simulink model "teleoperationTwoArm"  (R2012b)
settings: Solver=ode45  StartTime=0.0  StopTime=10  RelTol=1e-3
settings Model: Creator=aruszkowski  LastModifiedBy=davinci
settings DataIOCC: SignalLoggingSaveFormat=ModelDataLogs  SaveOutput=off  SaveTime=off
settings OptimizationCC: ExpressionDepthLimit=128
settings DebuggingCC: ReadBeforeWriteMsg=DisableAll  WriteAfterWriteMsg=DisableAll  WriteAfterReadMsg=DisableAll  MultiTaskDSMMsg=warning  MultiTaskCondExecSysMsg=none  StateNameClashWarn=none  StrictBusMsg=None
settings ModelReferenceCC: UpdateModelReferenceTargets=IfOutOfDate
settings SFSimCC: SFSimEcho=off
settings RTWCC: IncludeERTFirstTime=on
settings CodeAppCC: CustomSymbolStrType=$N$R$M_T  InternalIdentifier=Shortened

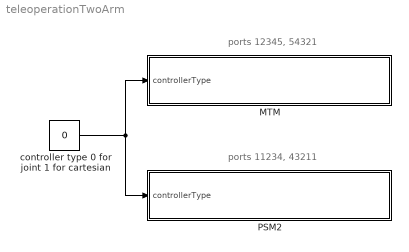
== system teleoperationTwoArm ==
  note: ports 12345, 54321
  note: ports 11234, 43211
  MTM : Subsystem
  PSM2 : Subsystem
  controller type 0 for joint 1 for cartesian : Constant  Value=0
  wires:
  controller type 0 for joint 1 for cartesian/1 -> PSM2/1(controllerType), MTM/1(controllerType)

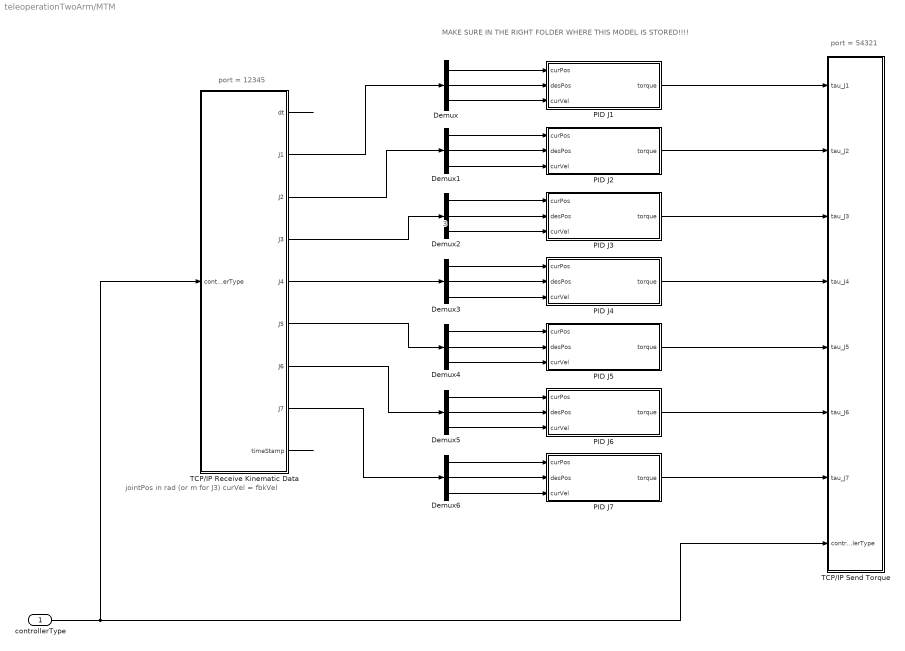
== system teleoperationTwoArm/MTM ==
  note: MAKE SURE IN THE RIGHT FOLDER WHERE THIS MODEL IS STORED!!!!
  note: port = 54321
  note: port = 12345
  note: 3
  note: jointPos in rad (or m for J3)
      | curVel = fbkVel
  controllerType : Inport
  Demux{,1..6} (7 alike) : Demux  Outputs=3
  PID J1 : Subsystem
  PID J2 : Subsystem
  PID J3 : Subsystem
  PID J4 : Subsystem
  PID J5 : Subsystem
  PID J6 : Subsystem
  PID J7 : Subsystem
  TCP/IP Receive Kinematic Data : Subsystem
  TCP/IP Send Torque : Subsystem  TreatAsAtomicUnit=on
  wires:
  TCP/IP Receive Kinematic Data/8(J7) -> Demux6/1
  Demux/1 -> PID J1/1(curPos)
  Demux/2 -> PID J1/2(desPos)
  Demux1/2 -> PID J2/2(desPos)
  Demux1/3 -> PID J2/3(curVel)
  Demux2/1 -> PID J3/1(curPos)
  PID J5/1(torque) -> TCP/IP Send Torque/5(tau_J5)
  PID J7/1(torque) -> TCP/IP Send Torque/7(tau_J7)
  controllerType/1 -> TCP/IP Receive Kinematic Data/1(controllerType), TCP/IP Send Torque/8(controllerType)
  TCP/IP Receive Kinematic Data/6(J5) -> Demux4/1
  TCP/IP Receive Kinematic Data/7(J6) -> Demux5/1
  Demux5/3 -> PID J6/3(curVel)
  Demux6/1 -> PID J7/1(curPos)
  TCP/IP Receive Kinematic Data/1(dt) -> ?
  TCP/IP Receive Kinematic Data/9(timeStamp) -> ?
  Demux6/2 -> PID J7/2(desPos)
  Demux4/3 -> PID J5/3(curVel)
  TCP/IP Receive Kinematic Data/2(J1) -> Demux/1
  Demux1/1 -> PID J2/1(curPos)
  Demux2/3 -> PID J3/3(curVel)
  Demux2/2 -> PID J3/2(desPos)
  TCP/IP Receive Kinematic Data/3(J2) -> Demux1/1
  Demux4/2 -> PID J5/2(desPos)
  Demux5/1 -> PID J6/1(curPos)
  Demux/3 -> PID J1/3(curVel)
  Demux5/2 -> PID J6/2(desPos)
  TCP/IP Receive Kinematic Data/4(J3) -> Demux2/1
  TCP/IP Receive Kinematic Data/5(J4) -> Demux3/1
  PID J2/1(torque) -> TCP/IP Send Torque/2(tau_J2)
  PID J4/1(torque) -> TCP/IP Send Torque/4(tau_J4)
  PID J3/1(torque) -> TCP/IP Send Torque/3(tau_J3)
  PID J1/1(torque) -> TCP/IP Send Torque/1(tau_J1)
  Demux6/3 -> PID J7/3(curVel)
  PID J6/1(torque) -> TCP/IP Send Torque/6(tau_J6)
  Demux3/3 -> PID J4/3(curVel)
  Demux4/1 -> PID J5/1(curPos)
  Demux3/1 -> PID J4/1(curPos)
  Demux3/2 -> PID J4/2(desPos)

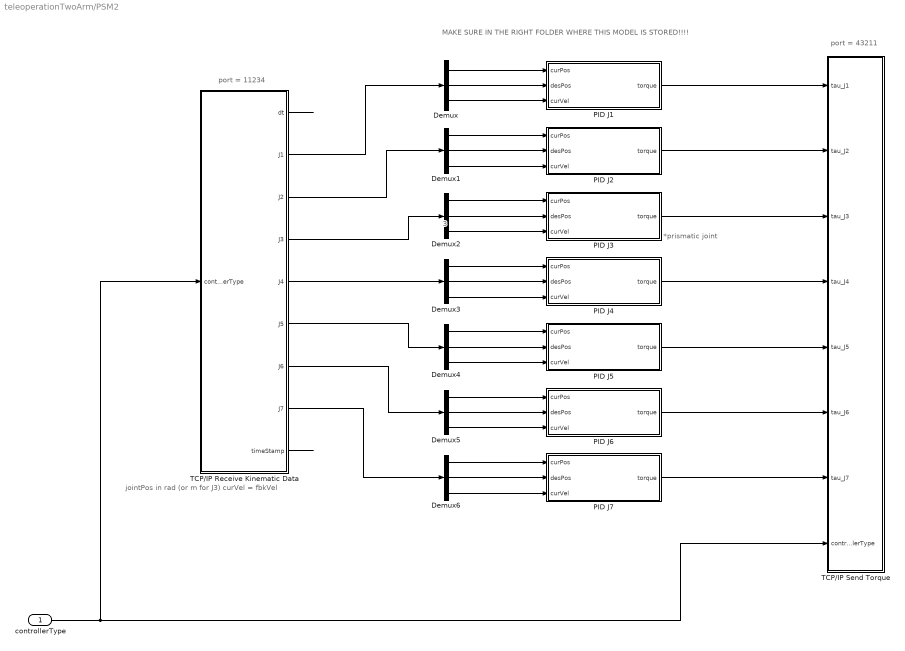
== system teleoperationTwoArm/PSM2 ==
  note: *prismatic joint
  note: jointPos in rad (or m for J3)
      | curVel = fbkVel
  note: 3
  note: port = 11234
  note: port = 43211
  note: MAKE SURE IN THE RIGHT FOLDER WHERE THIS MODEL IS STORED!!!!
  controllerType : Inport
  Demux{,1..6} (7 alike) : Demux  Outputs=3
  PID J1 : Subsystem
  PID J2 : Subsystem
  PID J3 : Subsystem
  PID J4 : Subsystem
  PID J5 : Subsystem
  PID J6 : Subsystem
  PID J7 : Subsystem
  TCP/IP Receive Kinematic Data : Subsystem
  TCP/IP Send Torque : Subsystem  TreatAsAtomicUnit=on
  wires:
  Demux3/2 -> PID J4/2(desPos)
  Demux3/1 -> PID J4/1(curPos)
  Demux4/1 -> PID J5/1(curPos)
  Demux3/3 -> PID J4/3(curVel)
  PID J6/1(torque) -> TCP/IP Send Torque/6(tau_J6)
  Demux6/3 -> PID J7/3(curVel)
  PID J1/1(torque) -> TCP/IP Send Torque/1(tau_J1)
  PID J3/1(torque) -> TCP/IP Send Torque/3(tau_J3)
  PID J4/1(torque) -> TCP/IP Send Torque/4(tau_J4)
  PID J2/1(torque) -> TCP/IP Send Torque/2(tau_J2)
  TCP/IP Receive Kinematic Data/5(J4) -> Demux3/1
  TCP/IP Receive Kinematic Data/4(J3) -> Demux2/1
  Demux5/2 -> PID J6/2(desPos)
  Demux/3 -> PID J1/3(curVel)
  Demux5/1 -> PID J6/1(curPos)
  Demux4/2 -> PID J5/2(desPos)
  TCP/IP Receive Kinematic Data/3(J2) -> Demux1/1
  Demux2/2 -> PID J3/2(desPos)
  Demux2/3 -> PID J3/3(curVel)
  Demux1/1 -> PID J2/1(curPos)
  TCP/IP Receive Kinematic Data/2(J1) -> Demux/1
  Demux4/3 -> PID J5/3(curVel)
  Demux6/2 -> PID J7/2(desPos)
  TCP/IP Receive Kinematic Data/9(timeStamp) -> ?
  TCP/IP Receive Kinematic Data/1(dt) -> ?
  Demux6/1 -> PID J7/1(curPos)
  Demux5/3 -> PID J6/3(curVel)
  TCP/IP Receive Kinematic Data/7(J6) -> Demux5/1
  TCP/IP Receive Kinematic Data/6(J5) -> Demux4/1
  controllerType/1 -> TCP/IP Send Torque/8(controllerType), TCP/IP Receive Kinematic Data/1(controllerType)
  PID J7/1(torque) -> TCP/IP Send Torque/7(tau_J7)
  PID J5/1(torque) -> TCP/IP Send Torque/5(tau_J5)
  Demux2/1 -> PID J3/1(curPos)
  Demux1/3 -> PID J2/3(curVel)
  Demux1/2 -> PID J2/2(desPos)
  Demux/2 -> PID J1/2(desPos)
  Demux/1 -> PID J1/1(curPos)
  TCP/IP Receive Kinematic Data/8(J7) -> Demux6/1

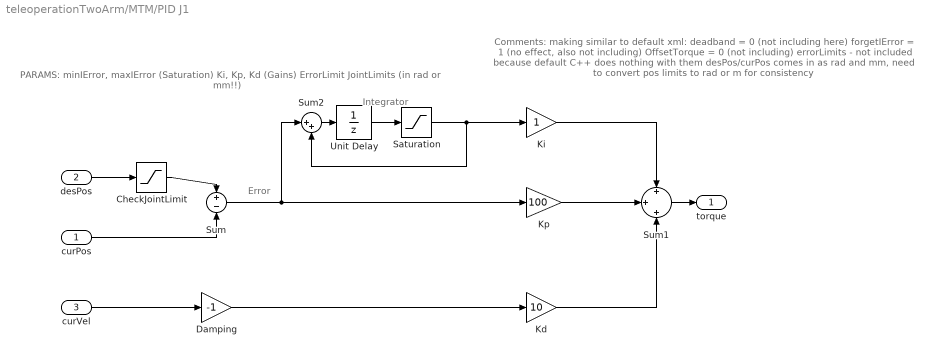
== system teleoperationTwoArm/MTM/PID J1 ==
  note: Error
  note: Comments: making similar to default xml:
      | deadband = 0 (not including here)
      | forgetIError = 1 (no effect, also not including)
      | OffsetTorque = 0 (not including)
      | errorLimits - not included because default C++ does nothing with them
      | desPos/curPos comes in as rad and mm, need to convert pos limits to rad or m for consistency
  note: PARAMS:
      | minIError, maxIError (Saturation)
      | Ki, Kp, Kd (Gains)
      | ErrorLimit
      | JointLimits (in rad or mm!!)
  note: Integrator
  curPos : Inport
  desPos : Inport  Port=2
  curVel : Inport  Port=3
  CheckJointLimit : Saturate  UpperLimit=70*pi()/180  LowerLimit=-40*pi()/180
  Damping : Gain  Gain=-1
  Kd : Gain  Gain=10
  Ki : Gain
  Kp : Gain  Gain=100
  Saturation : Saturate  UpperLimit=100  LowerLimit=-100  ZeroCross=off
  Sum : Sum  Inputs=+|-
  Sum1 : Sum  Inputs=+|+|+
  Sum2 : Sum  Inputs=|++
  Unit Delay : UnitDelay  SampleTime=-1
  torque : Outport
  wires:
  Saturation/1 -> Sum2/2, Ki/1
  Kp/1 -> Sum1/2
  Ki/1 -> Sum1/1
  Kd/1 -> Sum1/3
  CheckJointLimit/1 -> Sum/1
  desPos/1 -> CheckJointLimit/1
  Sum1/1 -> torque/1
  curPos/1 -> Sum/2
  curVel/1 -> Damping/1
  Damping/1 -> Kd/1
  Sum2/1 -> Unit Delay/1
  Unit Delay/1 -> Saturation/1
  Sum/1 -> Sum2/1, Kp/1

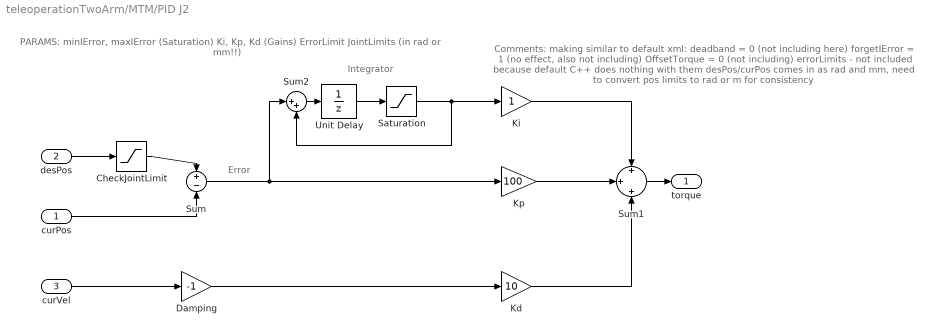
== system teleoperationTwoArm/MTM/PID J2 ==
  note: Error
  note: Integrator
  note: Comments: making similar to default xml:
      | deadband = 0 (not including here)
      | forgetIError = 1 (no effect, also not including)
      | OffsetTorque = 0 (not including)
      | errorLimits - not included because default C++ does nothing with them
      | desPos/curPos comes in as rad and mm, need to convert pos limits to rad or m for consistency
  note: PARAMS:
      | minIError, maxIError (Saturation)
      | Ki, Kp, Kd (Gains)
      | ErrorLimit
      | JointLimits (in rad or mm!!)
  curPos : Inport
  desPos : Inport  Port=2
  curVel : Inport  Port=3
  CheckJointLimit : Saturate  UpperLimit=65*pi()/180  LowerLimit=-20*pi()/180
  Damping : Gain  Gain=-1
  Kd : Gain  Gain=10
  Ki : Gain
  Kp : Gain  Gain=100
  Saturation : Saturate  UpperLimit=100  LowerLimit=-100  ZeroCross=off
  Sum : Sum  Inputs=+|-
  Sum1 : Sum  Inputs=+|+|+
  Sum2 : Sum  Inputs=|++
  Unit Delay : UnitDelay  SampleTime=-1
  torque : Outport
  wires:
  Kp/1 -> Sum1/2
  Ki/1 -> Sum1/1
  Kd/1 -> Sum1/3
  CheckJointLimit/1 -> Sum/1
  desPos/1 -> CheckJointLimit/1
  Sum1/1 -> torque/1
  curPos/1 -> Sum/2
  curVel/1 -> Damping/1
  Damping/1 -> Kd/1
  Saturation/1 -> Ki/1, Sum2/2
  Sum2/1 -> Unit Delay/1
  Unit Delay/1 -> Saturation/1
  Sum/1 -> Sum2/1, Kp/1

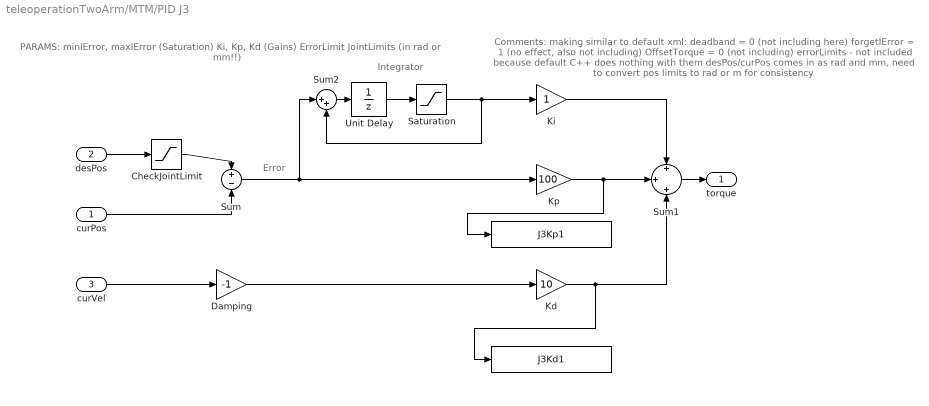
== system teleoperationTwoArm/MTM/PID J3 ==
  note: Error
  note: Comments: making similar to default xml:
      | deadband = 0 (not including here)
      | forgetIError = 1 (no effect, also not including)
      | OffsetTorque = 0 (not including)
      | errorLimits - not included because default C++ does nothing with them
      | desPos/curPos comes in as rad and mm, need to convert pos limits to rad or m for consistency
  note: PARAMS:
      | minIError, maxIError (Saturation)
      | Ki, Kp, Kd (Gains)
      | ErrorLimit
      | JointLimits (in rad or mm!!)
  note: Integrator
  curPos : Inport
  desPos : Inport  Port=2
  curVel : Inport  Port=3
  "      " : ToWorkspace  VariableName=J3Kp1  SampleTime=-1  SaveFormat=Timeseries
  "        " : ToWorkspace  VariableName=J3Kd1  SampleTime=-1  SaveFormat=Timeseries
  CheckJointLimit : Saturate  UpperLimit=35  LowerLimit=-50
  Damping : Gain  Gain=-1
  Kd : Gain  Gain=10
  Ki : Gain
  Kp : Gain  Gain=100
  Saturation : Saturate  UpperLimit=100  LowerLimit=-100  ZeroCross=off
  Sum : Sum  Inputs=+|-
  Sum1 : Sum  Inputs=+|+|+
  Sum2 : Sum  Inputs=|++
  Unit Delay : UnitDelay  SampleTime=-1
  torque : Outport
  wires:
  Kp/1 -> "      "/1, Sum1/2
  Ki/1 -> Sum1/1
  Kd/1 -> "        "/1, Sum1/3
  CheckJointLimit/1 -> Sum/1
  desPos/1 -> CheckJointLimit/1
  Sum1/1 -> torque/1
  curPos/1 -> Sum/2
  curVel/1 -> Damping/1
  Damping/1 -> Kd/1
  Saturation/1 -> Ki/1, Sum2/2
  Sum2/1 -> Unit Delay/1
  Unit Delay/1 -> Saturation/1
  Sum/1 -> Sum2/1, Kp/1

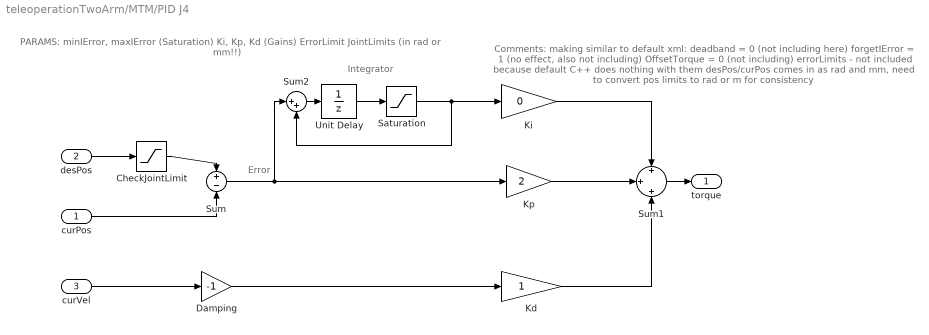
== system teleoperationTwoArm/MTM/PID J4 ==
  note: Error
  note: Integrator
  note: Comments: making similar to default xml:
      | deadband = 0 (not including here)
      | forgetIError = 1 (no effect, also not including)
      | OffsetTorque = 0 (not including)
      | errorLimits - not included because default C++ does nothing with them
      | desPos/curPos comes in as rad and mm, need to convert pos limits to rad or m for consistency
  note: PARAMS:
      | minIError, maxIError (Saturation)
      | Ki, Kp, Kd (Gains)
      | ErrorLimit
      | JointLimits (in rad or mm!!)
  curPos : Inport
  desPos : Inport  Port=2
  curVel : Inport  Port=3
  CheckJointLimit : Saturate  UpperLimit=90*pi()/180  LowerLimit=-200*pi()/180
  Damping : Gain  Gain=-1
  Kd : Gain
  Ki : Gain  Gain=0
  Kp : Gain  Gain=2
  Saturation : Saturate  UpperLimit=100  LowerLimit=-100  ZeroCross=off
  Sum : Sum  Inputs=+|-
  Sum1 : Sum  Inputs=+|+|+
  Sum2 : Sum  Inputs=|++
  Unit Delay : UnitDelay  SampleTime=-1
  torque : Outport
  wires:
  Kp/1 -> Sum1/2
  Ki/1 -> Sum1/1
  Kd/1 -> Sum1/3
  CheckJointLimit/1 -> Sum/1
  desPos/1 -> CheckJointLimit/1
  Sum1/1 -> torque/1
  curPos/1 -> Sum/2
  curVel/1 -> Damping/1
  Damping/1 -> Kd/1
  Saturation/1 -> Ki/1, Sum2/2
  Sum2/1 -> Unit Delay/1
  Unit Delay/1 -> Saturation/1
  Sum/1 -> Sum2/1, Kp/1

== system teleoperationTwoArm/MTM/PID J5 ==
  note: Error
  note: Comments: making similar to default xml:
      | deadband = 0 (not including here)
      | forgetIError = 1 (no effect, also not including)
      | OffsetTorque = 0 (not including)
      | errorLimits - not included because default C++ does nothing with them
      | desPos/curPos comes in as rad and mm, need to convert pos limits to rad or m for consistency
  note: PARAMS:
      | minIError, maxIError (Saturation)
      | Ki, Kp, Kd (Gains)
      | ErrorLimit
      | JointLimits (in rad or mm!!)
  note: Integrator
  curPos : Inport
  desPos : Inport  Port=2
  curVel : Inport  Port=3
  CheckJointLimit : Saturate  UpperLimit=180*pi()/180  LowerLimit=-90*pi()/180
  Damping : Gain  Gain=-1
  Kd : Gain
  Ki : Gain  Gain=0
  Kp : Gain  Gain=2
  Saturation : Saturate  UpperLimit=100  LowerLimit=-100  ZeroCross=off
  Sum : Sum  Inputs=+|-
  Sum1 : Sum  Inputs=+|+|+
  Sum2 : Sum  Inputs=|++
  Unit Delay : UnitDelay  SampleTime=-1
  torque : Outport
  wires:
  Kp/1 -> Sum1/2
  Ki/1 -> Sum1/1
  Kd/1 -> Sum1/3
  CheckJointLimit/1 -> Sum/1
  desPos/1 -> CheckJointLimit/1
  Sum1/1 -> torque/1
  curPos/1 -> Sum/2
  curVel/1 -> Damping/1
  Damping/1 -> Kd/1
  Saturation/1 -> Ki/1, Sum2/2
  Sum2/1 -> Unit Delay/1
  Unit Delay/1 -> Saturation/1
  Sum/1 -> Sum2/1, Kp/1

== system teleoperationTwoArm/MTM/PID J6 ==
  note: Error
  note: Integrator
  note: Comments: making similar to default xml:
      | deadband = 0 (not including here)
      | forgetIError = 1 (no effect, also not including)
      | OffsetTorque = 0 (not including)
      | errorLimits - not included because default C++ does nothing with them
      | desPos/curPos comes in as rad and mm, need to convert pos limits to rad or m for consistency
  note: PARAMS:
      | minIError, maxIError (Saturation)
      | Ki, Kp, Kd (Gains)
      | ErrorLimit
      | JointLimits (in rad or mm!!)
  curPos : Inport
  desPos : Inport  Port=2
  curVel : Inport  Port=3
  CheckJointLimit : Saturate  UpperLimit=40*pi()/180  LowerLimit=-45*pi()/180
  Damping : Gain  Gain=-1
  Kd : Gain
  Ki : Gain  Gain=0
  Kp : Gain  Gain=2
  Saturation : Saturate  UpperLimit=100  LowerLimit=-100  ZeroCross=off
  Sum : Sum  Inputs=+|-
  Sum1 : Sum  Inputs=+|+|+
  Sum2 : Sum  Inputs=|++
  Unit Delay : UnitDelay  SampleTime=-1
  torque : Outport
  wires:
  Kp/1 -> Sum1/2
  Ki/1 -> Sum1/1
  Kd/1 -> Sum1/3
  CheckJointLimit/1 -> Sum/1
  desPos/1 -> CheckJointLimit/1
  Sum1/1 -> torque/1
  curPos/1 -> Sum/2
  curVel/1 -> Damping/1
  Damping/1 -> Kd/1
  Saturation/1 -> Ki/1, Sum2/2
  Sum2/1 -> Unit Delay/1
  Unit Delay/1 -> Saturation/1
  Sum/1 -> Sum2/1, Kp/1

== system teleoperationTwoArm/MTM/PID J7 ==
  note: Error
  note: Comments: making similar to default xml:
      | deadband = 0 (not including here)
      | forgetIError = 1 (no effect, also not including)
      | OffsetTorque = 0 (not including)
      | errorLimits - not included because default C++ does nothing with them
      | desPos/curPos comes in as rad and mm, need to convert pos limits to rad or m for consistency
  note: PARAMS:
      | minIError, maxIError (Saturation)
      | Ki, Kp, Kd (Gains)
      | ErrorLimit
      | JointLimits (in rad or mm!!)
  note: Integrator
  curPos : Inport
  desPos : Inport  Port=2
  curVel : Inport  Port=3
  CheckJointLimit : Saturate  UpperLimit=180*pi()/180  LowerLimit=-180*pi()/180
  Damping : Gain  Gain=-1
  Kd : Gain  Gain=5
  Ki : Gain  Gain=0
  Kp : Gain
  Saturation : Saturate  UpperLimit=100  LowerLimit=-100  ZeroCross=off
  Sum : Sum  Inputs=+|-
  Sum1 : Sum  Inputs=+|+|+
  Sum2 : Sum  Inputs=|++
  Unit Delay : UnitDelay  SampleTime=-1
  torque : Outport
  wires:
  Kp/1 -> Sum1/2
  Ki/1 -> Sum1/1
  Kd/1 -> Sum1/3
  CheckJointLimit/1 -> Sum/1
  desPos/1 -> CheckJointLimit/1
  Sum1/1 -> torque/1
  curPos/1 -> Sum/2
  curVel/1 -> Damping/1
  Damping/1 -> Kd/1
  Saturation/1 -> Ki/1, Sum2/2
  Sum2/1 -> Unit Delay/1
  Unit Delay/1 -> Saturation/1
  Sum/1 -> Sum2/1, Kp/1

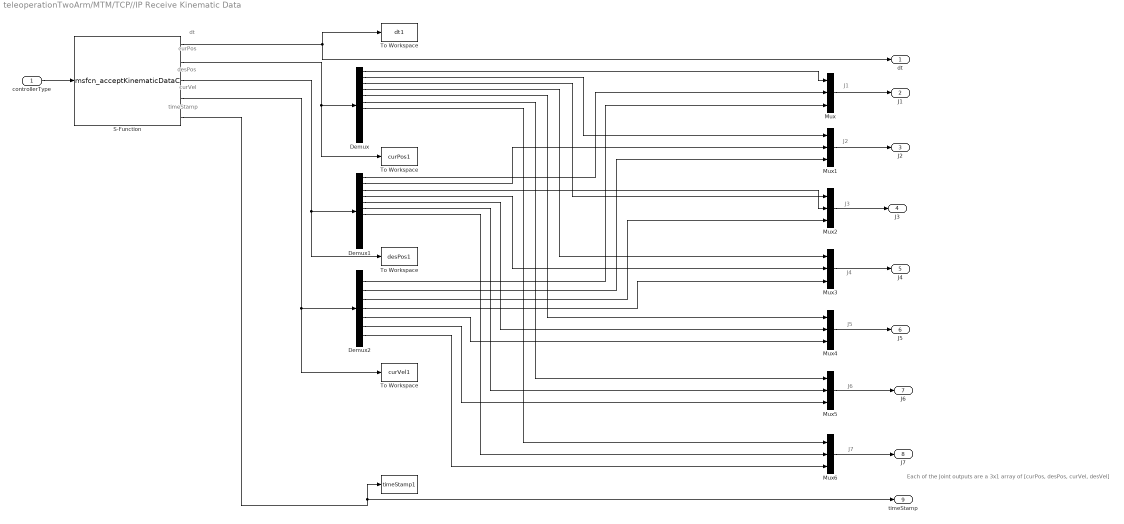
== system teleoperationTwoArm/MTM/TCP//IP Receive Kinematic Data ==
  note: timeStamp
  note: Each of the Joint outputs are a 3x1 array of
      | [curPos, desPos, curVel, desVel]
  note: J7
  note: J6
  note: J5
  note: J4
  note: J3
  note: J2
  note: J1
  note: curVel
  note: desPos
  note: curPos
  note: dt
  controllerType : Inport
  " " : ToWorkspace  VariableName=timeStamp1  SampleTime=-1  SaveFormat=Timeseries
  Demux : Demux  Outputs=12
  Demux1 : Demux  Outputs=12
  Demux2 : Demux  Outputs=7
  Mux{,1..6} (7 alike) : Mux  Inputs=3
  S-Function : S-Function  FunctionName=msfcn_acceptKinematicDataC  Parameters='137.82.56.245', '12345'  EnableBusSupport=off
  To Workspace : ToWorkspace  VariableName=curPos1  SampleTime=-1  SaveFormat=Timeseries
  "To Workspace " : ToWorkspace  VariableName=desPos1  SampleTime=-1  SaveFormat=Timeseries
  "To Workspace " : ToWorkspace  VariableName=curVel1  SampleTime=-1  SaveFormat=Timeseries
  "To Workspace " : ToWorkspace  VariableName=dt1  SampleTime=-1  SaveFormat=Timeseries
  dt : Outport
  J1 : Outport  Port=2
  J2 : Outport  Port=3
  J3 : Outport  Port=4
  J4 : Outport  Port=5
  J5 : Outport  Port=6
  J6 : Outport  Port=7
  J7 : Outport  Port=8
  timeStamp : Outport  Port=9
  wires:
  Mux3/1 -> J4/1
  Demux1/1 -> Mux/2
  S-Function/1 -> dt/1, "To Workspace "/1
  Demux/7 -> Mux6/1
  Demux2/7 -> Mux6/3
  Demux/4 -> Mux3/1
  Demux1/3 -> Mux2/2
  Demux/6 -> Mux5/1
  Demux2/1 -> Mux/3
  Mux6/1 -> J7/1
  Demux/2 -> Mux1/1
  S-Function/4 -> Demux2/1, "To Workspace "/1
  Demux1/2 -> Mux1/2
  Mux4/1 -> J5/1
  S-Function/3 -> "To Workspace "/1, Demux1/1
  Demux2/6 -> Mux5/3
  Demux1/6 -> Mux5/2
  Demux1/7 -> Mux6/2
  Demux1/4 -> Mux3/2
  Demux1/5 -> Mux4/2
  Demux2/2 -> Mux1/3
  Demux2/4 -> Mux3/3
  Demux2/5 -> Mux4/3
  Mux/1 -> J1/1
  Mux5/1 -> J6/1
  Mux2/1 -> J3/1
  Demux/3 -> Mux2/1
  Demux2/3 -> Mux2/3
  Mux1/1 -> J2/1
  Demux/1 -> Mux/1
  S-Function/2 -> To Workspace/1, Demux/1
  Demux/5 -> Mux4/1
  S-Function/5 -> " "/1, timeStamp/1
  controllerType/1 -> S-Function/1

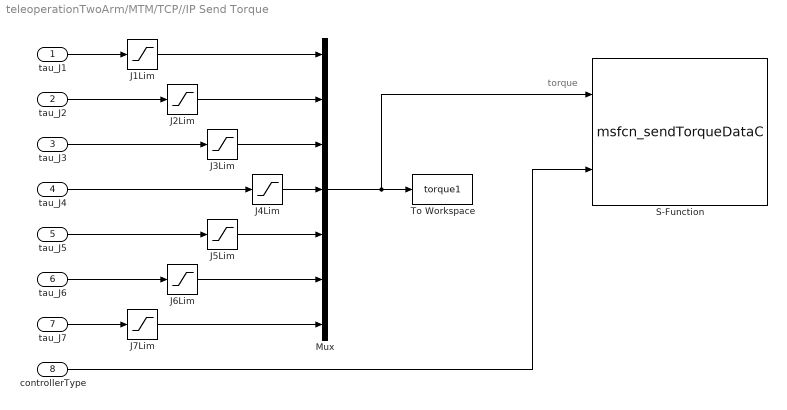
== system teleoperationTwoArm/MTM/TCP//IP Send Torque ==
  note: torque
  tau_J1 : Inport
  tau_J2 : Inport  Port=2
  tau_J3 : Inport  Port=3
  tau_J4 : Inport  Port=4
  tau_J5 : Inport  Port=5
  tau_J6 : Inport  Port=6
  tau_J7 : Inport  Port=7
  controllerType : Inport  Port=8
  J1Lim : Saturate  UpperLimit=900  LowerLimit=-900
  J2Lim : Saturate  UpperLimit=900  LowerLimit=-900
  J3Lim : Saturate  UpperLimit=900  LowerLimit=-900
  J4Lim : Saturate  UpperLimit=900  LowerLimit=-900
  J5Lim : Saturate  UpperLimit=900  LowerLimit=-900
  J6Lim : Saturate  UpperLimit=900  LowerLimit=-900
  J7Lim : Saturate  UpperLimit=900  LowerLimit=-900
  Mux : Mux  Inputs=7
  S-Function : S-Function  FunctionName=msfcn_sendTorqueDataC  Parameters='137.82.56.245', '54321'  EnableBusSupport=off
  To Workspace : ToWorkspace  VariableName=torque1  SampleTime=-1  SaveFormat=Timeseries
  wires:
  Mux/1 -> S-Function/1, To Workspace/1
  tau_J7/1 -> J7Lim/1
  tau_J6/1 -> J6Lim/1
  tau_J5/1 -> J5Lim/1
  tau_J4/1 -> J4Lim/1
  tau_J3/1 -> J3Lim/1
  tau_J2/1 -> J2Lim/1
  tau_J1/1 -> J1Lim/1
  J1Lim/1 -> Mux/1
  J2Lim/1 -> Mux/2
  J3Lim/1 -> Mux/3
  J5Lim/1 -> Mux/5
  J6Lim/1 -> Mux/6
  J7Lim/1 -> Mux/7
  J4Lim/1 -> Mux/4
  controllerType/1 -> S-Function/2

== system teleoperationTwoArm/PSM2/PID J1 ==
  note: Integrator
  note: PARAMS:
      | minIError, maxIError (Saturation)
      | Ki, Kp, Kd (Gains)
      | ErrorLimit
      | JointLimits (in rad or mm!!)
  note: Comments: making similar to default xml:
      | deadband = 0 (not including here)
      | forgetIError = 1 (no effect, also not including)
      | OffsetTorque = 0 (not including)
      | errorLimits - not included because default C++ does nothing with them
      | desPos/curPos comes in as rad and mm, need to convert pos limits to rad or m for consistency
  note: Error
  curPos : Inport
  desPos : Inport  Port=2
  curVel : Inport  Port=3
  CheckJointLimit : Saturate  UpperLimit=70*pi()/180  LowerLimit=-70*pi()/180
  Damping : Gain  Gain=-1
  Kd : Gain  Gain=5
  Ki : Gain  Gain=0
  Kp : Gain  Gain=50
  Saturation : Saturate  UpperLimit=20  LowerLimit=-20  ZeroCross=off
  Sum : Sum  Inputs=+|-
  Sum1 : Sum  Inputs=+|+|+
  Sum2 : Sum  Inputs=|++
  Unit Delay : UnitDelay  SampleTime=-1
  torque : Outport
  wires:
  Sum/1 -> Kp/1, Sum2/1
  Unit Delay/1 -> Saturation/1
  Sum2/1 -> Unit Delay/1
  Damping/1 -> Kd/1
  curVel/1 -> Damping/1
  curPos/1 -> Sum/2
  Sum1/1 -> torque/1
  desPos/1 -> CheckJointLimit/1
  CheckJointLimit/1 -> Sum/1
  Kd/1 -> Sum1/3
  Ki/1 -> Sum1/1
  Kp/1 -> Sum1/2
  Saturation/1 -> Ki/1, Sum2/2

== system teleoperationTwoArm/PSM2/PID J2 ==
  note: PARAMS:
      | minIError, maxIError (Saturation)
      | Ki, Kp, Kd (Gains)
      | ErrorLimit
      | JointLimits (in rad or mm!!)
  note: Comments: making similar to default xml:
      | deadband = 0 (not including here)
      | forgetIError = 1 (no effect, also not including)
      | OffsetTorque = 0 (not including)
      | errorLimits - not included because default C++ does nothing with them
      | desPos/curPos comes in as rad and mm, need to convert pos limits to rad or m for consistency
  note: Integrator
  note: Error
  curPos : Inport
  desPos : Inport  Port=2
  curVel : Inport  Port=3
  CheckJointLimit : Saturate  UpperLimit=50*pi()/180  LowerLimit=-50*pi()/180
  Damping : Gain  Gain=-1
  Kd : Gain  Gain=4
  Ki : Gain  Gain=0
  Kp : Gain  Gain=40
  Saturation : Saturate  UpperLimit=20  LowerLimit=-20  ZeroCross=off
  Sum : Sum  Inputs=+|-
  Sum1 : Sum  Inputs=+|+|+
  Sum2 : Sum  Inputs=|++
  Unit Delay : UnitDelay  SampleTime=-1
  torque : Outport
  wires:
  Sum/1 -> Kp/1, Sum2/1
  Unit Delay/1 -> Saturation/1
  Sum2/1 -> Unit Delay/1
  Saturation/1 -> Sum2/2, Ki/1
  Damping/1 -> Kd/1
  curVel/1 -> Damping/1
  curPos/1 -> Sum/2
  Sum1/1 -> torque/1
  desPos/1 -> CheckJointLimit/1
  CheckJointLimit/1 -> Sum/1
  Kd/1 -> Sum1/3
  Ki/1 -> Sum1/1
  Kp/1 -> Sum1/2

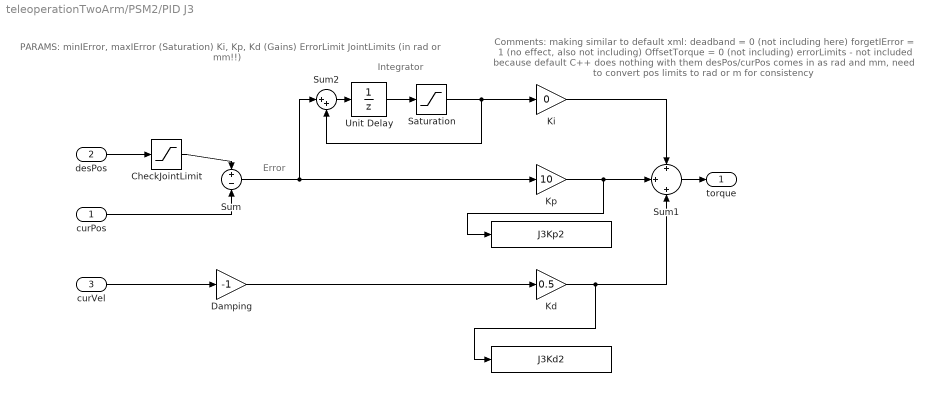
== system teleoperationTwoArm/PSM2/PID J3 ==
  note: Integrator
  note: PARAMS:
      | minIError, maxIError (Saturation)
      | Ki, Kp, Kd (Gains)
      | ErrorLimit
      | JointLimits (in rad or mm!!)
  note: Comments: making similar to default xml:
      | deadband = 0 (not including here)
      | forgetIError = 1 (no effect, also not including)
      | OffsetTorque = 0 (not including)
      | errorLimits - not included because default C++ does nothing with them
      | desPos/curPos comes in as rad and mm, need to convert pos limits to rad or m for consistency
  note: Error
  curPos : Inport
  desPos : Inport  Port=2
  curVel : Inport  Port=3
  "      " : ToWorkspace  VariableName=J3Kp2  SampleTime=-1  SaveFormat=Timeseries
  "        " : ToWorkspace  VariableName=J3Kd2  SampleTime=-1  SaveFormat=Timeseries
  CheckJointLimit : Saturate  UpperLimit=235  LowerLimit=0
  Damping : Gain  Gain=-1
  Kd : Gain  Gain=0.5
  Ki : Gain  Gain=0
  Kp : Gain  Gain=10
  Saturation : Saturate  UpperLimit=20  LowerLimit=-20  ZeroCross=off
  Sum : Sum  Inputs=+|-
  Sum1 : Sum  Inputs=+|+|+
  Sum2 : Sum  Inputs=|++
  Unit Delay : UnitDelay  SampleTime=-1
  torque : Outport
  wires:
  Sum/1 -> Kp/1, Sum2/1
  Unit Delay/1 -> Saturation/1
  Sum2/1 -> Unit Delay/1
  Saturation/1 -> Sum2/2, Ki/1
  Damping/1 -> Kd/1
  curVel/1 -> Damping/1
  curPos/1 -> Sum/2
  Sum1/1 -> torque/1
  desPos/1 -> CheckJointLimit/1
  CheckJointLimit/1 -> Sum/1
  Kd/1 -> Sum1/3, "        "/1
  Ki/1 -> Sum1/1
  Kp/1 -> Sum1/2, "      "/1

== system teleoperationTwoArm/PSM2/PID J4 ==
  note: PARAMS:
      | minIError, maxIError (Saturation)
      | Ki, Kp, Kd (Gains)
      | ErrorLimit
      | JointLimits (in rad or mm!!)
  note: Comments: making similar to default xml:
      | deadband = 0 (not including here)
      | forgetIError = 1 (no effect, also not including)
      | OffsetTorque = 0 (not including)
      | errorLimits - not included because default C++ does nothing with them
      | desPos/curPos comes in as rad and mm, need to convert pos limits to rad or m for consistency
  note: Integrator
  note: Error
  curPos : Inport
  desPos : Inport  Port=2
  curVel : Inport  Port=3
  CheckJointLimit : Saturate  UpperLimit=260*pi()/180  LowerLimit=-260*pi()/180
  Damping : Gain  Gain=-1
  Kd : Gain  Gain=0.05
  Ki : Gain  Gain=0.002
  Kp : Gain  Gain=0.5
  Saturation : Saturate  UpperLimit=10  LowerLimit=-10  ZeroCross=off
  Sum : Sum  Inputs=+|-
  Sum1 : Sum  Inputs=+|+|+
  Sum2 : Sum  Inputs=|++
  Unit Delay : UnitDelay  SampleTime=-1
  torque : Outport
  wires:
  Sum/1 -> Kp/1, Sum2/1
  Unit Delay/1 -> Saturation/1
  Sum2/1 -> Unit Delay/1
  Saturation/1 -> Sum2/2, Ki/1
  Damping/1 -> Kd/1
  curVel/1 -> Damping/1
  curPos/1 -> Sum/2
  Sum1/1 -> torque/1
  desPos/1 -> CheckJointLimit/1
  CheckJointLimit/1 -> Sum/1
  Kd/1 -> Sum1/3
  Ki/1 -> Sum1/1
  Kp/1 -> Sum1/2

== system teleoperationTwoArm/PSM2/PID J5 ==
  note: Integrator
  note: PARAMS:
      | minIError, maxIError (Saturation)
      | Ki, Kp, Kd (Gains)
      | ErrorLimit
      | JointLimits (in rad or mm!!)
  note: Comments: making similar to default xml:
      | deadband = 0 (not including here)
      | forgetIError = 1 (no effect, also not including)
      | OffsetTorque = 0 (not including)
      | errorLimits - not included because default C++ does nothing with them
      | desPos/curPos comes in as rad and mm, need to convert pos limits to rad or m for consistency
  note: Error
  curPos : Inport
  desPos : Inport  Port=2
  curVel : Inport  Port=3
  CheckJointLimit : Saturate  UpperLimit=80*pi()/180  LowerLimit=-80*pi()/180
  Damping : Gain  Gain=-1
  Kd : Gain  Gain=0.05
  Ki : Gain  Gain=0.002
  Kp : Gain  Gain=0.5
  Saturation : Saturate  UpperLimit=5  LowerLimit=-5  ZeroCross=off
  Sum : Sum  Inputs=+|-
  Sum1 : Sum  Inputs=+|+|+
  Sum2 : Sum  Inputs=|++
  Unit Delay : UnitDelay  SampleTime=-1
  torque : Outport
  wires:
  Sum/1 -> Kp/1, Sum2/1
  Unit Delay/1 -> Saturation/1
  Sum2/1 -> Unit Delay/1
  Saturation/1 -> Sum2/2, Ki/1
  Damping/1 -> Kd/1
  curVel/1 -> Damping/1
  curPos/1 -> Sum/2
  Sum1/1 -> torque/1
  desPos/1 -> CheckJointLimit/1
  CheckJointLimit/1 -> Sum/1
  Kd/1 -> Sum1/3
  Ki/1 -> Sum1/1
  Kp/1 -> Sum1/2

== system teleoperationTwoArm/PSM2/PID J6 ==
  note: PARAMS:
      | minIError, maxIError (Saturation)
      | Ki, Kp, Kd (Gains)
      | ErrorLimit
      | JointLimits (in rad or mm!!)
  note: Comments: making similar to default xml:
      | deadband = 0 (not including here)
      | forgetIError = 1 (no effect, also not including)
      | OffsetTorque = 0 (not including)
      | errorLimits - not included because default C++ does nothing with them
      | desPos/curPos comes in as rad and mm, need to convert pos limits to rad or m for consistency
  note: Integrator
  note: Error
  curPos : Inport
  desPos : Inport  Port=2
  curVel : Inport  Port=3
  CheckJointLimit : Saturate  UpperLimit=80*pi()/180  LowerLimit=-80*pi()/180
  Damping : Gain  Gain=-1
  Kd : Gain  Gain=0.05
  Ki : Gain  Gain=0.002
  Kp : Gain  Gain=0.5
  Saturation : Saturate  UpperLimit=5  LowerLimit=-5  ZeroCross=off
  Sum : Sum  Inputs=+|-
  Sum1 : Sum  Inputs=+|+|+
  Sum2 : Sum  Inputs=|++
  Unit Delay : UnitDelay  SampleTime=-1
  torque : Outport
  wires:
  Sum/1 -> Kp/1, Sum2/1
  Unit Delay/1 -> Saturation/1
  Sum2/1 -> Unit Delay/1
  Saturation/1 -> Sum2/2, Ki/1
  Damping/1 -> Kd/1
  curVel/1 -> Damping/1
  curPos/1 -> Sum/2
  Sum1/1 -> torque/1
  desPos/1 -> CheckJointLimit/1
  CheckJointLimit/1 -> Sum/1
  Kd/1 -> Sum1/3
  Ki/1 -> Sum1/1
  Kp/1 -> Sum1/2

== system teleoperationTwoArm/PSM2/PID J7 ==
  note: Integrator
  note: PARAMS:
      | minIError, maxIError (Saturation)
      | Ki, Kp, Kd (Gains)
      | ErrorLimit
      | JointLimits (in rad or mm!!)
  note: Comments: making similar to default xml:
      | deadband = 0 (not including here)
      | forgetIError = 1 (no effect, also not including)
      | OffsetTorque = 0 (not including)
      | errorLimits - not included because default C++ does nothing with them
      | desPos/curPos comes in as rad and mm, need to convert pos limits to rad or m for consistency
  note: Error
  curPos : Inport
  desPos : Inport  Port=2
  curVel : Inport  Port=3
  CheckJointLimit : Saturate  UpperLimit=80*pi()/180  LowerLimit=-80*pi()/180
  Damping : Gain  Gain=-1
  Kd : Gain  Gain=0.01
  Ki : Gain  Gain=0.003
  Kp : Gain  Gain=0.2
  Saturation : Saturate  UpperLimit=5  LowerLimit=-5  ZeroCross=off
  Sum : Sum  Inputs=+|-
  Sum1 : Sum  Inputs=+|+|+
  Sum2 : Sum  Inputs=|++
  Unit Delay : UnitDelay  SampleTime=-1
  torque : Outport
  wires:
  Sum/1 -> Kp/1, Sum2/1
  Unit Delay/1 -> Saturation/1
  Sum2/1 -> Unit Delay/1
  Saturation/1 -> Sum2/2, Ki/1
  Damping/1 -> Kd/1
  curVel/1 -> Damping/1
  curPos/1 -> Sum/2
  Sum1/1 -> torque/1
  desPos/1 -> CheckJointLimit/1
  CheckJointLimit/1 -> Sum/1
  Kd/1 -> Sum1/3
  Ki/1 -> Sum1/1
  Kp/1 -> Sum1/2

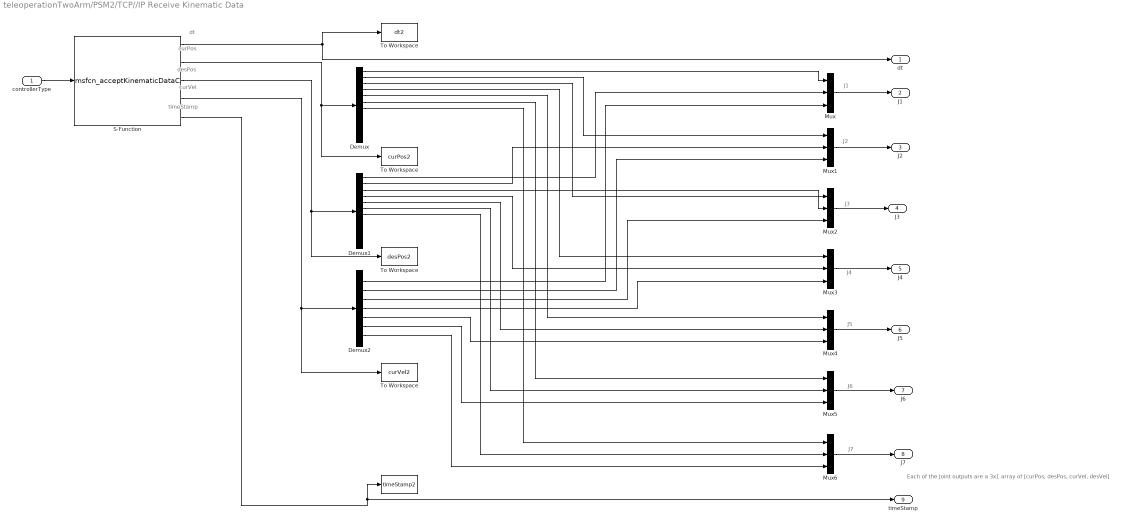
== system teleoperationTwoArm/PSM2/TCP//IP Receive Kinematic Data ==
  note: dt
  note: curPos
  note: desPos
  note: curVel
  note: J1
  note: J2
  note: J3
  note: J4
  note: J5
  note: J6
  note: J7
  note: Each of the Joint outputs are a 3x1 array of
      | [curPos, desPos, curVel, desVel]
  note: timeStamp
  controllerType : Inport
  " " : ToWorkspace  VariableName=timeStamp2  SampleTime=-1  SaveFormat=Timeseries
  Demux : Demux  Outputs=12
  Demux1 : Demux  Outputs=12
  Demux2 : Demux  Outputs=7
  Mux{,1..6} (7 alike) : Mux  Inputs=3
  S-Function : S-Function  FunctionName=msfcn_acceptKinematicDataC  Parameters='137.82.56.245', '11234'  EnableBusSupport=off
  To Workspace : ToWorkspace  VariableName=curPos2  SampleTime=-1  SaveFormat=Timeseries
  "To Workspace " : ToWorkspace  VariableName=desPos2  SampleTime=-1  SaveFormat=Timeseries
  "To Workspace " : ToWorkspace  VariableName=curVel2  SampleTime=-1  SaveFormat=Timeseries
  "To Workspace " : ToWorkspace  VariableName=dt2  SampleTime=-1  SaveFormat=Timeseries
  dt : Outport
  J1 : Outport  Port=2
  J2 : Outport  Port=3
  J3 : Outport  Port=4
  J4 : Outport  Port=5
  J5 : Outport  Port=6
  J6 : Outport  Port=7
  J7 : Outport  Port=8
  timeStamp : Outport  Port=9
  wires:
  controllerType/1 -> S-Function/1
  S-Function/5 -> timeStamp/1, " "/1
  Demux/5 -> Mux4/1
  S-Function/2 -> To Workspace/1, Demux/1
  Demux/1 -> Mux/1
  Mux1/1 -> J2/1
  Demux2/3 -> Mux2/3
  Demux/3 -> Mux2/1
  Mux2/1 -> J3/1
  Mux5/1 -> J6/1
  Mux/1 -> J1/1
  Demux2/5 -> Mux4/3
  Demux2/4 -> Mux3/3
  Demux2/2 -> Mux1/3
  Demux1/5 -> Mux4/2
  Demux1/4 -> Mux3/2
  Demux1/7 -> Mux6/2
  Demux1/6 -> Mux5/2
  Demux2/6 -> Mux5/3
  S-Function/3 -> Demux1/1, "To Workspace "/1
  Mux4/1 -> J5/1
  Demux1/2 -> Mux1/2
  S-Function/4 -> "To Workspace "/1, Demux2/1
  Demux/2 -> Mux1/1
  Mux6/1 -> J7/1
  Demux2/1 -> Mux/3
  Demux/6 -> Mux5/1
  Demux1/3 -> Mux2/2
  Demux/4 -> Mux3/1
  Demux2/7 -> Mux6/3
  Demux/7 -> Mux6/1
  S-Function/1 -> "To Workspace "/1, dt/1
  Demux1/1 -> Mux/2
  Mux3/1 -> J4/1

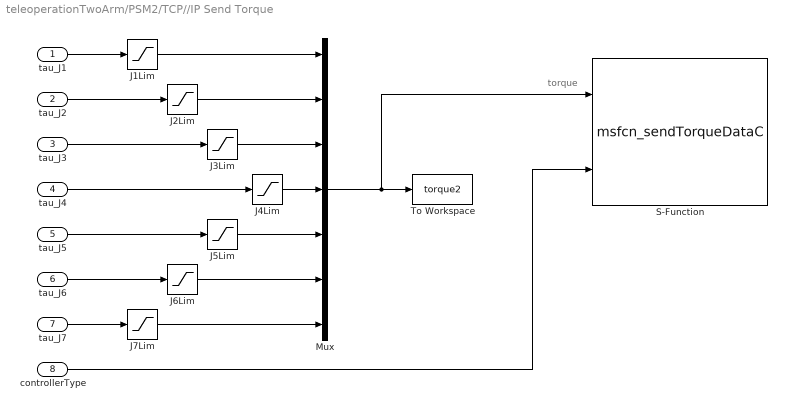
== system teleoperationTwoArm/PSM2/TCP//IP Send Torque ==
  note: torque
  tau_J1 : Inport
  tau_J2 : Inport  Port=2
  tau_J3 : Inport  Port=3
  tau_J4 : Inport  Port=4
  tau_J5 : Inport  Port=5
  tau_J6 : Inport  Port=6
  tau_J7 : Inport  Port=7
  controllerType : Inport  Port=8
  J1Lim : Saturate  UpperLimit=900  LowerLimit=-900
  J2Lim : Saturate  UpperLimit=900  LowerLimit=-900
  J3Lim : Saturate  UpperLimit=900  LowerLimit=-900
  J4Lim : Saturate  UpperLimit=900  LowerLimit=-900
  J5Lim : Saturate  UpperLimit=900  LowerLimit=-900
  J6Lim : Saturate  UpperLimit=900  LowerLimit=-900
  J7Lim : Saturate  UpperLimit=900  LowerLimit=-900
  Mux : Mux  Inputs=7
  S-Function : S-Function  FunctionName=msfcn_sendTorqueDataC  Parameters='137.82.56.245', '43211'  EnableBusSupport=off
  To Workspace : ToWorkspace  VariableName=torque2  SampleTime=-1  SaveFormat=Timeseries
  wires:
  controllerType/1 -> S-Function/2
  J4Lim/1 -> Mux/4
  J7Lim/1 -> Mux/7
  J6Lim/1 -> Mux/6
  J5Lim/1 -> Mux/5
  J3Lim/1 -> Mux/3
  J2Lim/1 -> Mux/2
  J1Lim/1 -> Mux/1
  tau_J1/1 -> J1Lim/1
  tau_J2/1 -> J2Lim/1
  tau_J3/1 -> J3Lim/1
  tau_J4/1 -> J4Lim/1
  tau_J5/1 -> J5Lim/1
  tau_J6/1 -> J6Lim/1
  tau_J7/1 -> J7Lim/1
  Mux/1 -> To Workspace/1, S-Function/1
